simulink model "Full_model"  (R2021a)
settings: Solver=VariableStepAuto  StartTime=0.0  StopTime=10.0  RelTol=1e-3
values from neighbouring files (symbols this model uses):
  L = 0.115    [Courant_matlab.m]
  r = 95.2*10^-3    (= 0.0952)    [dynamic_plaque.m]
  R = 3.6    [Courant_matlab.m]
settings Model: Creator=antho  LastModifiedBy=dupa1607

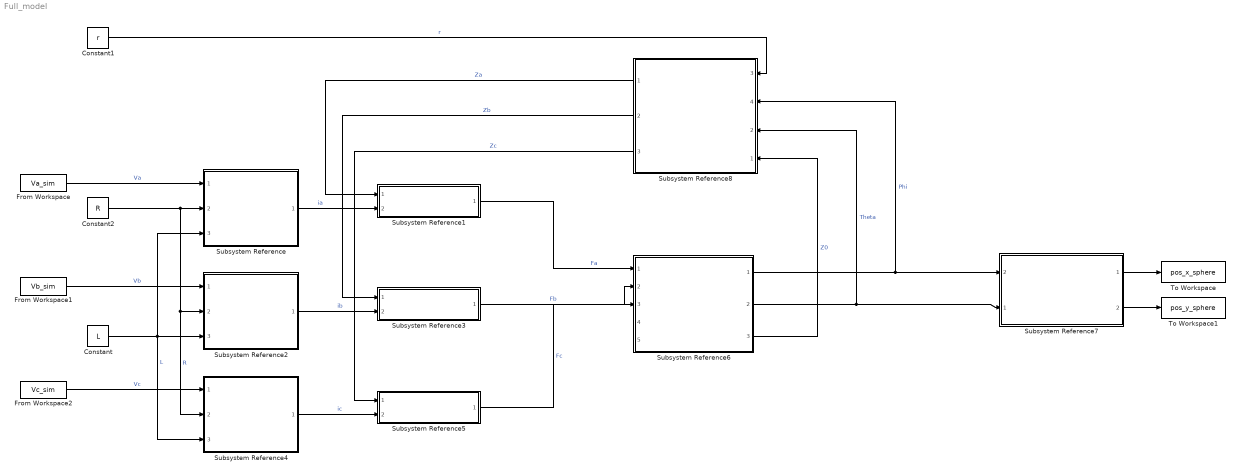
== system Full_model ==
  Constant : Constant  Value=L
  Constant1 : Constant  Value=r
  Constant2 : Constant  Value=R
  From Workspace : FromWorkspace  VariableName=Va_sim
  From Workspace1 : FromWorkspace  VariableName=Vb_sim
  From Workspace2 : FromWorkspace  VariableName=Vc_sim
  Subsystem Reference : Subsystem  ReferencedSubsystem=subsys_courant
  Subsystem Reference1 : Subsystem  ReferencedSubsystem=subsys_force
  Subsystem Reference2 : Subsystem  ReferencedSubsystem=subsys_courant
  Subsystem Reference3 : Subsystem  ReferencedSubsystem=subsys_force
  Subsystem Reference4 : Subsystem  ReferencedSubsystem=subsys_courant
  Subsystem Reference5 : Subsystem  ReferencedSubsystem=subsys_force
  Subsystem Reference6 : Subsystem  ReferencedSubsystem=subsys_dynamic_plaque
  Subsystem Reference7 : Subsystem  ReferencedSubsystem=subsys_sphere_position
      settings: PortSchema="{\"entries\":[{\"content\":{\"sides\":[{\"content\":{\"connectorIds\":[\"In2\",\"In1\"]},\"type\":\"ConnectorPlacement.EquallySpacedRectSide\",\"uuid\":\"96a04a08-4352-43c8-a8bd-dce0633e76dd\"},{\"content\":{\"connectorIds\":[\"Out1\",\"Out2\"],\"side\":\"RIGHT\"},\"type\":\"ConnectorPlacement.EquallySpacedRectSide\",\"uuid\":\"6371aec0-efd7-4766-a972-236c23c9f028\"},{\"content\":{\"connectorIds\":[],\"side\":\"TOP\"},\"type\":\"ConnectorPlacement.EquallySpacedRectSide\",\"uuid\":\"d707f900-e5a5-42aa-a3e1-854061b3e5bc\"}]},\"type\":\"ConnectorPlacement.EquallySpacedConnector\",\"uuid\":\"29279e07-6ad8-4183-91e5-486e6736f1f9\"}],\"packageUris\":[\"http://schema.mathworks.com/mf0/Connector/R2020b\"],\"version\":\"1.0\"}"
  Subsystem Reference8 : Subsystem  ReferencedSubsystem=subsys_hauteur_aimants
      settings: PortSchema="{\"entries\":[{\"content\":{\"sides\":[{\"content\":{\"connectorIds\":[\"In3\",\"In4\",\"In2\",\"In1\"]},\"type\":\"ConnectorPlacement.EquallySpacedRectSide\",\"uuid\":\"aad0297c-2a16-40e4-ae4d-ded4810484bd\"},{\"content\":{\"connectorIds\":[\"Out1\",\"Out2\",\"Out3\"],\"side\":\"RIGHT\"},\"type\":\"ConnectorPlacement.EquallySpacedRectSide\",\"uuid\":\"a548181b-8d4f-4e8c-8e81-e157a1504375\"},{\"content\":{\"connectorIds\":[],\"side\":\"TOP\"},\"type\":\"ConnectorPlacement.EquallySpacedRectSide\",\"uuid\":\"36d9bd6e-86ec-486f-98ec-c4e19d794fba\"}]},\"type\":\"ConnectorPlacement.EquallySpacedConnector\",\"uuid\":\"cbff7459-b836-4b55-8a47-eadd2f910e6f\"}],\"packageUris\":[\"http://schema.mathworks.com/mf0/Connector/R2020b\"],\"version\":\"1.0\"}"
  To Workspace : ToWorkspace  VariableName=pos_x_sphere  SaveFormat=Timeseries  SampleTime=-1
  To Workspace1 : ToWorkspace  VariableName=pos_y_sphere  SaveFormat=Timeseries  SampleTime=-1
  wires:
  Subsystem Reference/1 -> Subsystem Reference1/2  "ia"
  Subsystem Reference2/1 -> Subsystem Reference3/2  "ib"
  Subsystem Reference4/1 -> Subsystem Reference5/2  "ic"
  Subsystem Reference1/1 -> Subsystem Reference6/1  "Fa"
  Subsystem Reference3/1 -> Subsystem Reference6/2  "Fb"
  Subsystem Reference5/1 -> Subsystem Reference6/3  "Fc"
  Subsystem Reference6/2 -> Subsystem Reference8/2, Subsystem Reference7/1  "Theta"
  Subsystem Reference6/1 -> Subsystem Reference8/4, Subsystem Reference7/2  "Phi"
  Subsystem Reference6/3 -> Subsystem Reference8/1  "Z0"
  Subsystem Reference8/1 -> Subsystem Reference1/1  "Za"
  Subsystem Reference8/2 -> Subsystem Reference3/1  "Zb"
  Subsystem Reference8/3 -> Subsystem Reference5/1  "Zc"
  Constant1/1 -> Subsystem Reference8/3  "r"
  Constant/1 -> Subsystem Reference/3, Subsystem Reference4/3, Subsystem Reference2/3  "L"
  Constant2/1 -> Subsystem Reference4/2, Subsystem Reference2/2, Subsystem Reference/2  "R"
  From Workspace/1 -> Subsystem Reference/1  "Va"
  Subsystem Reference7/2 -> To Workspace1/1
  Subsystem Reference7/1 -> To Workspace/1
  From Workspace1/1 -> Subsystem Reference2/1  "Vb"
  From Workspace2/1 -> Subsystem Reference4/1  "Vc"
